simulink model "Wind_AC_PLL_22a"  (R2022a)
settings: Solver=ode23t  StartTime=0.0  StopTime=Setpoint.PLL.Tsim  RelTol=1e-3
undefined symbols (not defined in the file or in its folder): Electric, Generator, Plate, R_h2, Setpoint
libraries: fl_lib x36, nesl_utility x17, ee_lib x15, spsRMSLib x1
(part 4 of 4)

== matlab function Wind_AC_PLL_22a/Electrolyzer/Sensor/MATLAB Function ==
  data: u input; Z output
function Z = fcn(u)

Z = min(u(2)/u(1),1e3);
